simulink model "model"  (R2025a)
settings: Solver=VariableStepAuto  StartTime=0.0  StopTime=20  MaxStep=0.002  RelTol=1e-3
libraries: slpidlib x1
settings Model: Creator=noast  LastModifiedBy=noast

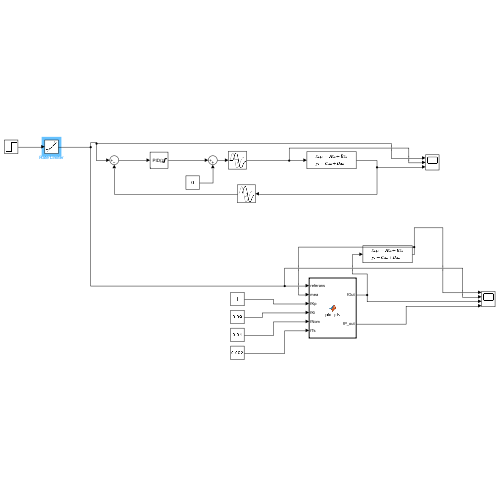
[thumbnail: Simulink's stored preview of the top-level diagram]
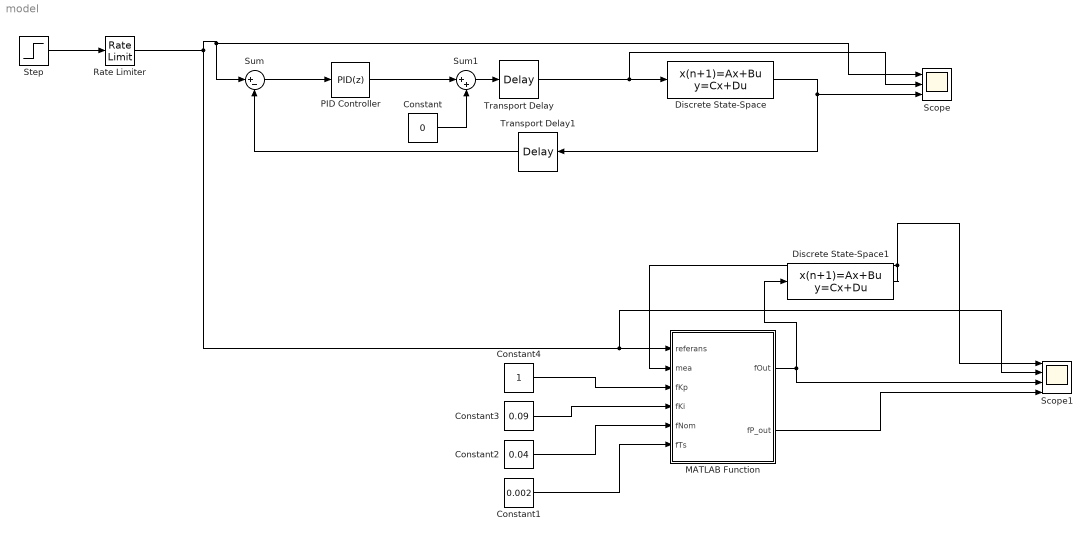
== system model ==
  Constant : Constant  Value=0
  Constant1 : Constant  Value=0.002
  Constant2 : Constant  Value=0.04
  Constant3 : Constant  Value=0.09
  Constant4 : Constant
  Discrete State-Space : DiscreteStateSpace  A=0.999841  B=0.001587  D=0  InitialCondition=0.4  SampleTime=-1
  Discrete State-Space1 : DiscreteStateSpace  A=0.999841  B=0.001587  D=0  InitialCondition=0.4  SampleTime=-1
  MATLAB Function : MATLAB Function  TreatAsAtomicUnit=on
  PID Controller : slpidlib/PID Controller  Controller=PID  Form=Parallel  TimeDomain=Discrete-time  UseExternalTs=off  SampleTime=-1  IntegratorMethod=Forward Euler  FilterMethod=Forward Euler  ControllerParametersSource=internal  P=5  I=0.09  UseKiTs=off  D=0  UseExternalDerivativeSource=off  N=100  UseFilter=on  TunerSelectOption=Transfer Function Based (PID Tuner App)  InitialConditionSource=internal  InitialConditionForIntegrator=0.04  InitialConditionForFilter=0  DifferentiatorICPrevScaledInput=0  ExternalReset=none  TrackingMode=off  Kt=1  LimitOutput=on  SatLimitsSource=internal  UpperSaturationLimit=inf  LowerSaturationLimit=-inf  LinearizeAsGain=on  AntiWindupMode=back-calculation  Kb=1  LimitIntegrator=off  UpperIntegratorSaturationLimit=inf  LowerIntegratorSaturationLimit=-inf  POutMin=[]  POutMax=[]  IOutMin=[]  IOutMax=[]  DOutMin=[]  DOutMax=[]  NOutMin=[]  NOutMax=[]  SumOutMin=[]  SumOutMax=[]  SaturationOutMin=[]  SaturationOutMax=[]  PParamMin=[]  PParamMax=[]  IParamMin=[]  IParamMax=[]  DParamMin=[]  DParamMax=[]  NParamMin=[]  NParamMax=[]  KbParamMin=[]  KbParamMax=[]  KtParamMin=[]  KtParamMax=[]  KbOutMin=[]  KbOutMax=[]  KtOutMin=[]  KtOutMax=[]  IntegratorOutMin=[]  IntegratorOutMax=[]  FilterOutMin=[]  FilterOutMax=[]  SumI1OutMin=[]  SumI1OutMax=[]  SumI2OutMin=[]  SumI2OutMax=[]  SumI3OutMin=[]  SumI3OutMax=[]  SumI4OutMin=[]  SumI4OutMax=[]  SumDOutMin=[]  SumDOutMax=[]  DifferentiatorOutMin=[]  DifferentiatorOutMax=[]  FilterDiffOutCoefMin=[]  FilterDiffOutCoefMax=[]  ReciprocalOutMin=[]  ReciprocalOutMax=[]  SumDenOutMin=[]  SumDenOutMax=[]  SumNumOutMin=[]  SumNumOutMax=[]  DivideOutMin=[]  DivideOutMax=[]  UdiffTsProdOutMin=[]  UdiffTsProdOutMax=[]  NTsProdOutMin=[]  NTsProdOutMax=[]  UintegralTsProdOutMin=[]  UintegralTsProdOutMax=[]  UngainTsProdOutMin=[]  UngainTsProdOutMax=[]  ClampingZeroOutDataTypeStr=Inherit: Inherit via back propagation  ClampingZeroOutMin=[]  ClampingZeroOutMax=[]  FilterDenConstantOutDataTypeStr=Inherit: Inherit via back propagation  FilterDenConstantOutMin=[]  FilterDenConstantOutMax=[]  PCopyOutDataTypeStr=Inherit: Inherit via back propagation  PCopyOutMin=[]  PCopyOutMax=[]  NCopyOutDataTypeStr=Inherit: Inherit via back propagation  NCopyOutMin=[]  NCopyOutMax=[]  IntegratorContinuousStateAttributes=''  IntegratorStateMustResolveToSignalObject=off  IntegratorRTWStateStorageClass=Auto  FilterContinuousStateAttributes=''  FilterStateMustResolveToSignalObject=off  FilterRTWStateStorageClass=Auto  ParallelPVariant=InternalParameters  IdealPVariant=Disabled  IVariant=InternalParameters  DVariant=InternalParameters  IntegratorVariant=Discrete  SatVariant=Enabled  AWVariant=BackCalculation  PCopyVariant=Disabled  TRVariant=Disabled  FdbkBlocksVariant=Forward  IdealPFdbkVariant=Disabled  SatFdbkVariant=Disabled  DerivativeFilterVariant=ForwardEulerFilter  NVariant=InternalParameters  NCopyVariant=Disabled  FilterICVariant=InternalICsFilter  IntegratorICVariant=InternalICs  ExternalResetVariant=Disabled  TRSumVariant=Passthrough  SumFdbkVariant=Disabled  SumVariant=Sum_PID  TsampFilterVariant=InternalTs  TsampNgainVariant=Passthrough  TsampIntegralVariant=Disabled_SignalSpec  ExternalSaturationOutDataTypeStr=Inherit: Same as second input  DerivativeSourceVariant=ErrorSignal  PreIntVariant=InternalPreInt
  Rate Limiter : RateLimiter  RisingSlewLimit=0.1  FallingSlewLimit=-0.1  SampleTimeMode=inherited
  Scope : Scope  NumInputPorts=3
      settings: ActiveDisplayYMinimum=-0.06326554840397372  ActiveDisplayYMaximum=0.56938993563576357
  Scope1 : Scope  NumInputPorts=4
      settings: ActiveDisplayYMinimum=-0.01757993357227236  ActiveDisplayYMaximum=0.55821940215045129
  Step : Step  Before=0.4  After=0.5  SampleTime=0
  Sum : Sum  Inputs=|+-
  Sum1 : Sum  Inputs=|++
  Transport Delay : TransportDelay  DelayTime=0.02
  Transport Delay1 : TransportDelay  DelayTime=0.02  InitialOutput=0.4
  wires:
  Transport Delay/1 -> Scope/2, Discrete State-Space/1
  Sum/1 -> PID Controller/1
  Discrete State-Space/1 -> Transport Delay1/1, Scope/3
  Rate Limiter/1 -> Scope1/2, MATLAB Function/1(referans), Scope/1, Sum/1
  PID Controller/1 -> Sum1/1
  Constant/1 -> Sum1/2
  Discrete State-Space1/1 -> Scope1/1, MATLAB Function/2(mea)
  MATLAB Function/1(fOut) -> Scope1/3, Discrete State-Space1/1
  MATLAB Function/2(fP_out) -> Scope1/4
  Constant4/1 -> MATLAB Function/3(fKp)
  Constant3/1 -> MATLAB Function/4(fKi)
  Constant2/1 -> MATLAB Function/5(fNom)
  Constant1/1 -> MATLAB Function/6(fTs)
  Sum1/1 -> Transport Delay/1
  Transport Delay1/1 -> Sum/2
  Step/1 -> Rate Limiter/1

== matlab function model/MATLAB Function ==
  data: referans input; fOut output; mea input; fKp input; fKi input; fNom input; fTs input; fP_out output
function [fOut, fP_out] = pid_pls(referans, mea, fKp, fKi, fNom, fTs)

persistent fI;
if isempty(fI)
    fI = fNom;  % = 4.0, samme som PLS
end

fError = double(referans) - mea;

% P-ledd
fP_out = fKp * fError;

% I-ledd
if fKi > 0.0
    fI = fI + fTs * fKi * fError;
else
    fI = fNom;
end

% Output
fRawOut = fP_out + fI;

% Begrens
if fRawOut > 100.0
    fOut = 100.0;
elseif fRawOut < 0.0
    fOut = 0.0;
else
    fOut = fRawOut;
end
